simulink model "LQG_test"  (R2016b)
settings: Solver=ode5  StartTime=0.0  StopTime=25  FixedStep=1e-4  RelTol=1e-3  EnableMultiTasking=on
values from neighbouring files (symbols this model uses):
  Ak = [-684.448289528 -1838.02275685 -245.449466562 329.096259703 75.0041195994 3.82706915823 1217.45439277 -372.514986285 172.466831781 194.781937877 259.855231872 9.91843311764 ... (36 elements, 6x6)]    [all_vars.mat]    (also in controller.mat; main_matlab.m = rlqg.A)
  Ap = [-19.7190772882 -1190.48104562 -62.676843111 18.0054766364 22.2223105278 -2.64108364066 1303.93904998 4.34224517238 -44.461064018 -131.114730905 -18.2113409342 5.33205678573 ... (36 elements, 6x6)]    [all_vars.mat]    (also in main_matlab.m = A; plant.mat)
  Bk = [-81.4819421286  292.924842313; 300.719243091  42.9479523448; -1170.07972993  -732.159461163; 254.772556959  876.819017487; -390.775314978  123.207611647; -45.8372700719  -43.6955248003]    [all_vars.mat]    (also in controller.mat; main_matlab.m = rlqg.B)
  Bp = [-7.24609198041  66.9700392934; -21.5039305656  73.576926911; 23.4984283525  21.403882812; 46.6827265176  -40.9539920145; 0.658674407167  -14.4888804429; 4.89041453042  0.290127980263]    [all_vars.mat]    (also in main_matlab.m = B; plant.mat)
  Ck = [1.54009703707  -0.116962618999  -2.09402947011  -5.28066592983  -1.24392730196  -9.20557682957; -8.80971369205  -3.43163961296  -5.78337983754  7.01971817871  -0.897914006953  -9.71423447702]    [all_vars.mat]    (also in controller.mat; main_matlab.m = rlqg.C)
  Cp = [-0.137816192394  0.472624836927  -0.0138484663098  0.0769834201517  -0.197522828123  0.399593591236; 0.178725450202  -0.354952725033  -0.223001269946  0.269122602377  0.582190972534  -0.765470552205]    [all_vars.mat]    (also in main_matlab.m = C; plant.mat)
  Dk = [0  0; 0  0]    [all_vars.mat]    (also in controller.mat; main_matlab.m = rlqg.D)
  Hp = [-4.79448602969 -1.99144171717 -19.445356322 -14.2821080896 0.877016765577 -1.80479844935]    [all_vars.mat]    (also in main_matlab.m = H; plant.mat)
libraries: simulink x1
settings Model: Creator=p4wp4w  LastModifiedBy=ABLAH
settings DataIOCC: LimitDataPoints=on  SaveFormat=Array
settings OptimizationCC: LifeSpan=inf
settings DebuggingCC: SFUnexpectedBacktrackingDiag=warning  SFNoUnconditionalDefaultTransitionDiag=warning  SFExecutionAtInitializationDiag=none
settings HardwareCC: ProdBitPerPointer=32  ProdBitPerSizeT=32  ProdBitPerPtrDiffT=32  ProdLargestAtomicFloat=None  ProdIntDivRoundTo=Undefined  ProdEndianess=Unspecified  ProdWordSize=32  ProdHWDeviceType=32-bit Generic
settings ModelReferenceCC: PropagateSignalLabelsOutOfModel=off
settings GRTTargetCC: TargetLangStandard=C89/C90 (ANSI)  GeneratePreprocessorConditionals=Disable all
settings ConfigComp: CovMetricSettings=dw  CovHtmlReporting=on  CovSaveCumulativeToWorkspaceVar=on  CovSaveSingleToWorkspaceVar=on  CovExternalEMLEnable=off

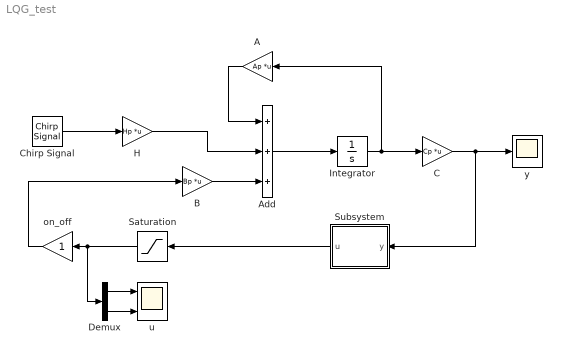
== system LQG_test ==
  A : Gain  Gain=Ap  Multiplication=Matrix(K*u)
  Add : Sum  Inputs=+++
  B : Gain  Gain=Bp  Multiplication=Matrix(K*u)
  C : Gain  Gain=Cp  Multiplication=Matrix(K*u)
  Chirp Signal : simulink/Sources/Chirp Signal  f1=0.1  T=25  f2=250
  Demux : Demux  Outputs=2
  H : Gain  Gain=Hp  Multiplication=Matrix(K*u)
  Integrator : Integrator
  Saturation : Saturate  UpperLimit=5  LowerLimit=-5
  Subsystem : Subsystem
  on_off : Gain
  u : Scope  NumInputPorts=2
  y : Scope
  wires:
  Add/1 -> Integrator/1
  A/1 -> Add/1
  B/1 -> Add/3
  Integrator/1 -> C/1, A/1
  H/1 -> Add/2
  Chirp Signal/1 -> H/1
  on_off/1 -> B/1
  Demux/1 -> u/1
  Demux/2 -> u/2
  Saturation/1 -> Demux/1, on_off/1
  C/1 -> Subsystem/1(y), y/1
  Subsystem/1("u ") -> Saturation/1

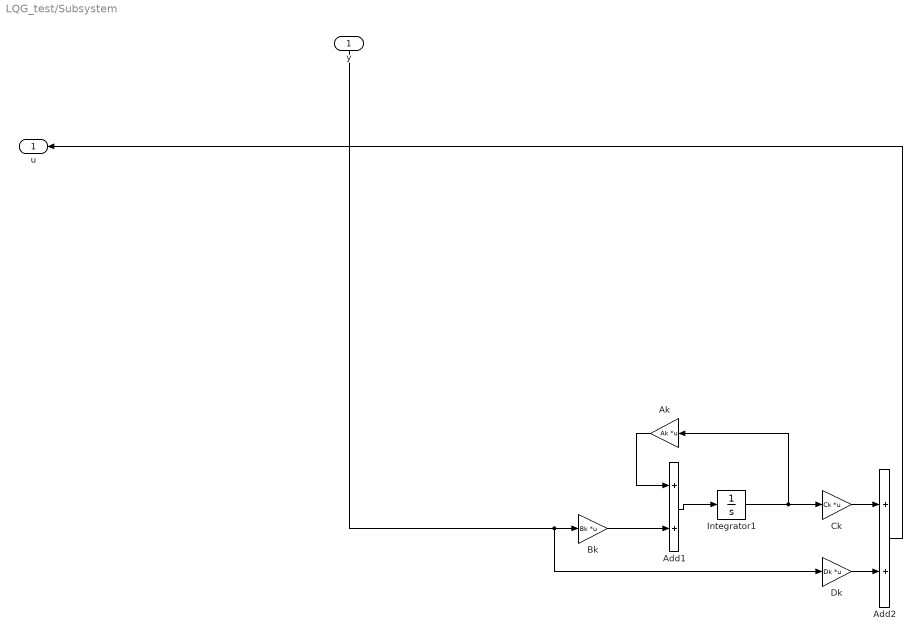
== system LQG_test/Subsystem ==
  y : Inport
  Add1 : Sum
  Add2 : Sum
  Ak : Gain  Gain=Ak  Multiplication=Matrix(K*u)
  Bk : Gain  Gain=Bk  Multiplication=Matrix(K*u)
  Ck : Gain  Gain=Ck  Multiplication=Matrix(K*u)
  Dk : Gain  Gain=Dk  Multiplication=Matrix(K*u)
  Integrator1 : Integrator
  "u " : Outport
  wires:
  y/1 -> Bk/1, Dk/1
  Add2/1 -> "u "/1
  Bk/1 -> Add1/2
  Ak/1 -> Add1/1
  Add1/1 -> Integrator1/1
  Dk/1 -> Add2/2
  Integrator1/1 -> Ck/1, Ak/1
  Ck/1 -> Add2/1
